simulink model "sim_mpc_lmi"  (Simulink 7.9)
settings: Solver=ode4  SolverMode=SingleTasking  StartTime=0.0  StopTime=10  FixedStep=0.01  RelTol=1e-3
undefined symbols (not defined in the file): A, Ac, B, Bc, C, T
settings Model: Creator=Kawakami  LastModifiedBy=Kawakami
settings DataIOCC: LimitDataPoints=off  SaveOutput=off  SaveTime=off  TimeSaveName=t  SignalLoggingName=sigsOut
settings OptimizationCC: BooleanDataType=off
settings DebuggingCC: SaveWithParameterizedLinksMsg=none  SignalResolutionControl=TryResolveAllWithWarning  SolverPrmCheckMsg=none  MultiTaskDSMMsg=warning  MultiTaskCondExecSysMsg=none  FcnCallInpInsideContextMsg=Use local settings  StrictBusMsg=None
settings HardwareCC: TargetUnknown=on
settings RTWCC: IncludeERTFirstTime=on
settings GRTTargetCC: CombineOutputUpdateFcns=off  GRTInterface=on

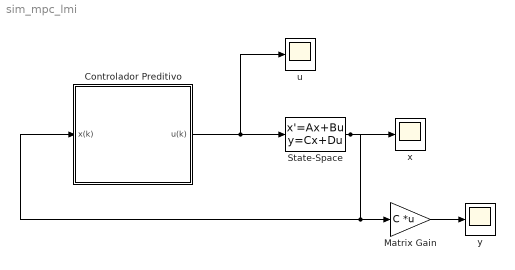
== system sim_mpc_lmi ==
  "Controlador Preditivo  " : Subsystem  mask{A=A, B=B, C=C, S=[1 0;0 1], R=1, umax=1*10, ymax=0.5*10, T=T}
  Matrix Gain : Gain  Gain=C  Multiplication=Matrix(K*u)  SaturateOnIntegerOverflow=on  OutDataTypeStr=Inherit: Same as input  ParamDataTypeStr=Inherit: Same as input
  State-Space : StateSpace  A=Ac  B=Bc  C=eye(size(Ac,1))  D=zeros(size(Ac,1),size(Bc,2))  X0=[2;1]
  u : Scope
      settings: TimeRange=10  YMin=-2  YMax=0.5
  x : Scope
      settings: YMin=-1.25  YMax=2.25
  y : Scope
      settings: TimeRange=10  YMin=-1  YMax=1  SaveName=ScopeData2
  wires:
  "Controlador Preditivo  "/1(u(k)) -> State-Space/1, u/1
  State-Space/1 -> x/1, "Controlador Preditivo  "/1(x(k)), Matrix Gain/1
  Matrix Gain/1 -> y/1

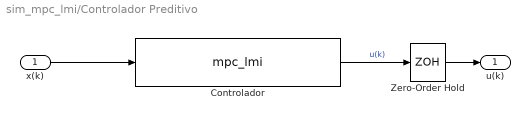
== system sim_mpc_lmi/Controlador Preditivo   ==
  x(k) : Inport
  Controlador : S-Function  FunctionName=mpc_lmi  Parameters=S,R,A,B,C,umax,ymax,T  EnableBusSupport=off
  Zero-Order Hold : ZeroOrderHold  SampleTime=T
  u(k) : Outport
  wires:
  Zero-Order Hold/1 -> u(k)/1
  Controlador/1 -> Zero-Order Hold/1  "u(k)"
  x(k)/1 -> Controlador/1
